simulink library "ddm"  (R2021b)
settings: Solver=VariableStepAuto  StartTime=0.0  StopTime=10.0  RelTol=1e-3
undefined symbols (not defined in the file or in its folder): ADDM_FrTMTqDev_X_Nm, ADDM_RrTMTqDev_X_Nm, ENUM_ADASACCSTA_ERROR, ENUM_ADASACCSTA_OFF, ENUM_ADASACCSTA_STANDBY, ENUM_ALLOWMOV_ALLOWREADY, ENUM_APS, ENUM_BRKSTA_ERROR, ENUM_BRKSTA_OFF, ENUM_BRKSTA_ON, ENUM_BRKSW_INVALID, ENUM_BRKSW_OFF, ENUM_BRKSW_ON, ENUM_CHGPREACTERRSTA_OBCPRE, ENUM_DCDCFAULTSTA_ANYFAULTLV1, ENUM_DCDCFAULTSTA_ANYFAULTLV2, ENUM_DRIVETRAIN_AWD, ENUM_DRIVETRAIN_FWD, ENUM_DRIVETRAIN_RWD, ENUM_EDUDRTSTA_NORMAL, ENUM_EPBSTA_APPLIED, ENUM_EPBSTA_RELEASED, ENUM_GEARACTUALPOSN_INVALID, ENUM_GEARACTUALPOSN_P, ENUM_HVBATTREADYPRE_READY, ENUM_MCUWARN_LV0, ENUM_MCUWARN_LV1, ENUM_MCUWARN_LV2, ENUM_MCUWARN_LV3, ENUM_MCUWARN_NOERROR, ENUM_OBCFAULTSTA_ANYFAULT, ENUM_PAS_R2F2, ENUM_PDFAULT_BATTPDFAIL, ENUM_PDFAULT_DCDCDISABLE, ENUM_PDFAULT_MCUDISABLE, ENUM_PDFAULT_MCUDISCHRG, ENUM_POWERSTA_OFF, ENUM_POWERSTA_ON, ENUM_POWERSTA_READY, ENUM_POWERSTA_STANDBY, ENUM_PRESSINDI_LOW, ENUM_PUFAULT_BATTUPFAIL, ENUM_PUFAULT_DCDCENABLEFAIL, ENUM_PUFAULT_PRECHRGCHKFAIL, ENUM_PUFAULT_SAFETYCHKFAIL, ENUM_PUSTATE_COMPLETED, ENUM_PWRSTASW_OFF, ENUM_PWRSTASW_OFFA, ENUM_PWRSTASW_OFFCHVCHRG, ENUM_PWRSTASW_OFFCLVCHRG, ENUM_PWRSTASW_ON, ENUM_PWRSTASW_ONHVCHRG, ENUM_PWRSTASW_READY, ENUM_PWRSTASW_STANDBY, ENUM_SHIFTCOMMAND_P, ENUM_SHIFTERERRSTA_PBUTTONFAILURE, ENUM_VEHMALFUNLV_2ND, ENUM_VEHMALFUNLV_3RD, ENUM_VEHMALFUNLV_4TH, ENUM_VEHMALFUNLV_NORMAL ... (+459)
libraries: hcu_lib x515, simulink x3
(part 21 of 25)

== system ddm/DDM/DDM/PMM/SW failure/Tailgate switch failure ==
  note: Diagnostics and Fault Handling
  note: Release Condition After Decision
  note: Test Detection Criteria
  note: Test Pass Criteria
  task_time_s : Inport
  VPMM_PowerSta_enum : Inport  Port=2
  VPMM_PwrStaSW_enum : Inport  Port=3
  VINP_TailgaSW : Inport  Port=4
  DTC_clear_request : Inport  Port=5
  Constant1 : Constant  Value=KDDM_TailgaSWDTC_cnt
  Constant11 : Constant  Value=KDDM_TailgaSWPassTO_s
  Constant12 : Constant  Value=ENUM_POWERSTA_STANDBY
  Constant13 : Constant  Value=ZERO_INT
  Constant15 : Constant  Value=KDDM_TailgaSWPassTO_s
  Constant16 : Constant  Value=KDDM_TailgaSWDetTO_s
  Constant17 : Constant  Value=KDDM_TailgaSW_s
  Constant18 : Constant  Value=FALSE
  Constant19 : Constant  Value=ENUM_PWRSTASW_OFF
  Constant2 : Constant  Value=KDDM_SWFailDiagnosisOffSW_flg
  Constant21 : Constant  Value=ZERO_INT
  Constant22 : Constant  Value=ENUM_PWRSTASW_OFF
  Constant23 : Constant  Value=TRUE
  Constant24 : Constant  Value=KDDM_TailgaSWPassTO_s
  Constant25 : Constant  Value=KDDM_TailgaSWDTC_cnt
  Constant26 : Constant  Value=ONE_INT
  Constant3 : Constant  Value=FALSE
  Constant32 : Constant  Value=ZERO_FLOAT
  Constant33 : Constant  Value=ENUM_POWERSTA_OFF
  Constant4 : Constant  Value=TRUE
  DTC_Couter2 : hcu_lib/Basic_Blocks/DTC_Couter
  DTC_Info : hcu_lib/Basic_Blocks/DTC_Info
  Data Type Conversion12 : DataTypeConversion  OutDataTypeStr=boolean
  Data Type Conversion14 : DataTypeConversion  OutDataTypeStr=boolean
  Data Type Conversion7 : DataTypeConversion
  Equal1 : RelationalOperator  Operator=~=  OutDataTypeStr=boolean  RndMeth=Simplest
  Equal11 : RelationalOperator  Operator===  OutDataTypeStr=boolean  RndMeth=Simplest
  Equal12 : RelationalOperator  Operator===  OutDataTypeStr=boolean  RndMeth=Simplest
  Equal3 : RelationalOperator  Operator=~=  OutDataTypeStr=boolean  RndMeth=Simplest
  Equal4 : RelationalOperator  Operator=~=  OutDataTypeStr=boolean  RndMeth=Simplest
  Equal5 : RelationalOperator  OutDataTypeStr=boolean  RndMeth=Simplest
  Logical Operator14 : Logic  Operator=OR  Inputs=4  AllPortsSameDT=off  OutDataTypeStr=boolean
  Logical Operator16 : Logic  AllPortsSameDT=off  OutDataTypeStr=boolean
  Logical Operator4 : Logic  Operator=NOT  AllPortsSameDT=off  OutDataTypeStr=boolean
  Logical Operator5 : Logic  Operator=NOT  AllPortsSameDT=off  OutDataTypeStr=boolean
  Logical Operator6 : Logic  AllPortsSameDT=off  OutDataTypeStr=boolean
  Logical Operator7 : Logic  Operator=NOT  AllPortsSameDT=off  OutDataTypeStr=boolean
  Relational Operator1 : RelationalOperator  Operator=>  OutDataTypeStr=boolean  RndMeth=Simplest
  Relational Operator4 : RelationalOperator  Operator=<=  OutDataTypeStr=boolean  RndMeth=Simplest
  Relational Operator5 : RelationalOperator  Operator=>  OutDataTypeStr=boolean  RndMeth=Simplest
  SR_Latch1 : hcu_lib/Basic_Blocks/SR_Latch
  Subsystem : Subsystem  AncestorBlock=ddm1/DDM/DDM/PMM/SW failure/Driver seat switch failure/Subsystem
  Switch{1,5,10,14} (4 alike) : Switch  Criteria=u2 ~= 0
  Terminator : Terminator
  Test Detection Criteria2 : hcu_lib/Basic_Blocks/Test Detection Criteria
  Timer : hcu_lib/Basic_Blocks/Test Detection Criteria/Timer
  Timer1 : hcu_lib/Basic_Blocks/Timer
  Unit Delay : UnitDelay  SampleTime=-1  HasFrameUpgradeWarning=on
  Unit Delay1 : UnitDelay  SampleTime=-1  HasFrameUpgradeWarning=on
  Unit Delay9 : UnitDelay  SampleTime=-1  HasFrameUpgradeWarning=on
  VDDM_TailgaSWDTC_raw32 : Outport
  VDDM_VCUTailgateSWSta_flg : Outport  Port=2
  VDDM_TailgaSWCFS_flg : Outport  Port=3
  wires:
  Switch1/1 -> VDDM_VCUTailgateSWSta_flg/1  "VDDM_VCUTailgateSWSta_flg"
  Constant3/1 -> Switch1/3
  [VDDM_TailgaSWCFS_flg] -> VDDM_TailgaSWCFS_flg/1, Switch1/2
  Constant4/1 -> Switch1/1
  Logical Operator14/1 -> [VDDM_TailgaSWCFSRls_flg]  "VDDM_TailgaSWCFSRls_flg"
  [VDDM_TailgaSWPass_flg] -> Logical Operator14/3
  Constant1/1 -> DTC_Couter2/3
  Relational Operator1/1 -> Terminator/1  "VDDM_TailgaSWDFS_flg"
  DTC_Couter2/2 -> Relational Operator1/1  "VDDM_TailgaSWDTC_cnt"
  Equal12/1 -> Logical Operator16/2
  DTC_Couter2/1 -> [VDDM_TailgaSWCFS_flg]  "VDDM_TailgaSWCFS_flg"
  Logical Operator16/1 -> Logical Operator14/1
  Equal11/1 -> Logical Operator16/1
  Constant13/1 -> Relational Operator1/2
  Constant2/1 -> Logical Operator14/4
  Constant12/1 -> Equal12/2
  [VDDM_TailgaSWCFSRls_flg] -> DTC_Couter2/2
  Unit Delay1/1 -> Equal11/1
  [DTC_clear_request] -> Logical Operator14/2
  Constant33/1 -> Equal11/2
  [VPMM_PowerSta_enum] -> Equal12/1
  [VPMM_PowerSta_enum] -> Unit Delay1/1
  [VDDM_TailgaSWDet_flg] -> DTC_Couter2/1
  Equal4/1 -> [VDDM_TailgaSWChange_flg]
  Data Type Conversion12/1 -> Test Detection Criteria2/1
  Subsystem/1(Fault_flg) -> Logical Operator6/1
  [VDDM_TailgaSWChange_flg] -> SR_Latch1/2
  Logical Operator7/1 -> Timer1/1
  [TailgaSWFault_flg] -> Switch10/1
  Data Type Conversion7/1 -> Test Detection Criteria2/4
  Test Detection Criteria2/1 -> [VDDM_TailgaSWDet_flg]  "VDDM_TailgaSWDet_flg"
  Constant26/1 -> SR_Latch1/1
  Switch5/1 -> Data Type Conversion12/1
  Constant32/1 -> Relational Operator5/2
  Switch10/1 -> Timer1/2, Logical Operator7/1
  Logical Operator6/1 -> Switch14/1, [TailgaSWFault_flg]
  [VPMM_PwrStaSW_enum] -> Equal1/1
  Relational Operator4/1 -> Logical Operator6/2
  [task_time_s] -> Timer1/3
  [task_time_s] -> Timer/3
  Constant21/1 -> Switch14/3
  Constant22/1 -> Equal1/2
  Data Type Conversion14/1 -> Equal4/1
  SR_Latch1/1 -> Timer/1, Logical Operator4/1, Logical Operator5/1
  Constant23/1 -> Switch10/3
  Logical Operator5/1 -> Subsystem/Trigger
  Constant17/1 -> Relational Operator4/2
  Constant24/1 -> Equal5/2
  [VINP_TailgaSWGPIO_flg] -> Relational Operator5/1
  Constant11/1 -> Timer/4
  Unit Delay/1 -> Subsystem/1(In1)
  Logical Operator4/1 -> Timer/2
  Relational Operator5/1 -> Equal4/2, Unit Delay9/1
  [task_time_s] -> Test Detection Criteria2/2
  [VDDM_TailgaSWCFSRls_flg] -> Switch5/2
  Constant18/1 -> Switch5/1
  Constant25/1 -> Test Detection Criteria2/3
  Equal5/1 -> [VDDM_TailgaSWPass_flg]  "VDDM_TailgaSWPass_flg"
  Timer1/1 -> Equal5/1
  Constant16/1 -> Data Type Conversion7/1
  Timer/1 -> Unit Delay/1, Relational Operator4/1
  Constant15/1 -> Timer1/4
  Unit Delay9/1 -> Data Type Conversion14/1
  Equal3/1 -> Switch10/2
  Switch14/1 -> Switch5/3
  Equal1/1 -> Switch14/2
  [VPMM_PwrStaSW_enum] -> Equal3/1
  Constant19/1 -> Equal3/2
  DTC_clear_request/1 -> [DTC_clear_request]
  VINP_TailgaSW/1 -> [VINP_TailgaSWGPIO_flg]
  task_time_s/1 -> [task_time_s]
  VPMM_PwrStaSW_enum/1 -> [VPMM_PwrStaSW_enum]
  VPMM_PowerSta_enum/1 -> [VPMM_PowerSta_enum]
  DTC_Info/1 -> VDDM_TailgaSWDTC_raw32/1  "VDDM_TailgaSWDTC_raw32"
  [VDDM_TailgaSWPass_flg] -> DTC_Info/2
  [VDDM_TailgaSWCFS_flg] -> DTC_Info/3
  [VDDM_TailgaSWDet_flg] -> DTC_Info/1
  [DTC_clear_request] -> DTC_Info/4

== system ddm/DDM/DDM/PMM/power up and power down/BMS HV relay closed fail ==
  note: Test Detection Criteria
  note: Test Pass Criteria
  note: Diagnostics and Fault Handling
  note: Release Condition After Decision
  task_time_s : Inport
  VPMM_PowerSta_enum : Inport  Port=2
  VPMM_PwrStaSW_enum : Inport  Port=3
  VINP_HVBContactorSta_flg : Inport  Port=4
  VPMM_PowerUpFault_enum : Inport  Port=5
  DTC_clear_request : Inport  Port=6
  VPMM_PowerUpState_enum : Inport  Port=7
  Constant : Constant  Value=ENUM_PUFAULT_BATTUPFAIL
  Constant12 : Constant  Value=ENUM_PWRSTASW_OFF
  Constant13 : Constant  Value=FALSE
  Constant14 : Constant  Value=ZERO_INT
  Constant17 : Constant  Value=KDDM_PwrUpDnDiagnosisOffSW_flg
  Constant18 : Constant  Value=KDDM_HVRlyCloDTC_cnt
  Constant22 : Constant  Value=ENUM_POWERSTA_OFF
  Constant28 : Constant  Value=KDDM_HVRlyCloDTC_cnt
  Constant29 : Constant  Value=FALSE
  Constant3 : Constant  Value=KDDM_HVRlyCloPassTO_s
  Constant4 : Constant  Value=FALSE
  Constant41 : Constant  Value=KDDM_HVRlyCloDetTO_s
  Constant5 : Constant  Value=ENUM_PUSTATE_COMPLETED
  Constant6 : Constant  Value=TRUE
  Constant7 : Constant  Value=ENUM_POWERSTA_STANDBY
  Constant9 : Constant  Value=KDDM_HVRlyCloPassTO_s
  DTC_Couter1 : hcu_lib/Basic_Blocks/DTC_Couter
  DTC_Info : hcu_lib/Basic_Blocks/DTC_Info
  Equal{1,3,8..9} (4 alike) : RelationalOperator  Operator===  OutDataTypeStr=boolean  RndMeth=Simplest
  Equal4 : RelationalOperator  Operator=~=  OutDataTypeStr=boolean  RndMeth=Simplest
  Equal7 : RelationalOperator  OutDataTypeStr=boolean  RndMeth=Simplest
  Logical Operator13 : Logic  Operator=NOT  AllPortsSameDT=off  OutDataTypeStr=boolean
  Logical Operator14 : Logic  Operator=OR  Inputs=4  AllPortsSameDT=off  OutDataTypeStr=boolean
  Logical Operator16 : Logic  AllPortsSameDT=off  OutDataTypeStr=boolean
  Logical Operator4 : Logic  Operator=NOT  AllPortsSameDT=off  OutDataTypeStr=boolean
  Logical Operator5 : Logic  AllPortsSameDT=off  OutDataTypeStr=boolean
  Relational Operator1 : RelationalOperator  Operator=>  OutDataTypeStr=boolean  RndMeth=Simplest
  Switch1 : Switch  Criteria=u2 ~= 0
  Switch3 : Switch  Criteria=u2 ~= 0
  Switch6 : Switch  Criteria=u2 ~= 0
  Terminator : Terminator
  Test Detection Criteria1 : hcu_lib/Basic_Blocks/Test Detection Criteria
  Timer2 : hcu_lib/Basic_Blocks/Timer
  Unit Delay1 : UnitDelay  SampleTime=-1  HasFrameUpgradeWarning=on
  VDDM_HVRlyCloDTC_raw32 : Outport
  VDDM_HVRlyCloCFS_flg : Outport  Port=2
  wires:
  [VDDM_HVRlyCloCFS_flg] -> VDDM_HVRlyCloCFS_flg/1
  DTC_Couter1/1 -> [VDDM_HVRlyCloCFS_flg]  "VDDM_HVRlyCloCFS_flg"
  [VPMM_PwrStaSW_enum] -> Equal4/1
  Equal7/1 -> [VDDM_HVRlyCloPass_flg]  "VDDM_HVRlyCloPass_flg"
  [task_time_s] -> Test Detection Criteria1/2
  Constant28/1 -> Test Detection Criteria1/3
  Unit Delay1/1 -> Equal8/1
  [VDDM_HVRlyCloChk_flg] -> Switch3/1
  Test Detection Criteria1/1 -> [VDDM_HVRlyCloDet_flg]  "VDDM_HVRlyCloDet_flg"
  Equal9/1 -> Logical Operator16/2
  DTC_Couter1/2 -> Relational Operator1/1  "VDDM_HVRlyCloDTC_cnt"
  Switch6/1 -> Test Detection Criteria1/1
  Constant3/1 -> Timer2/4
  Constant5/1 -> Equal3/2
  Switch1/1 -> Logical Operator13/1, Timer2/2
  Logical Operator14/1 -> [VDDM_HVRlyCloCFSRls_flg]  "VDDM_HVRlyCloCFSRls_flg"
  Switch3/1 -> Switch6/3
  Constant6/1 -> Switch1/3
  Constant13/1 -> Switch3/3
  Constant14/1 -> Relational Operator1/2
  [VDDM_HVRlyCloPass_flg] -> Logical Operator14/3
  [DTC_clear_request] -> Logical Operator14/2
  Constant29/1 -> Switch6/1
  Equal4/1 -> Switch3/2
  Constant9/1 -> Equal7/2
  [VDDM_HVRlyCloCFSRls_flg] -> DTC_Couter1/2
  Constant41/1 -> Test Detection Criteria1/4
  Logical Operator16/1 -> Logical Operator14/1
  Constant12/1 -> Equal4/2
  Logical Operator13/1 -> Timer2/1
  Equal8/1 -> Logical Operator16/1
  Equal3/1 -> Switch1/2
  [VPMM_PowerUpState_enum] -> Equal3/1
  Timer2/1 -> Equal7/1
  Constant18/1 -> DTC_Couter1/3
  Constant17/1 -> Logical Operator14/4
  [VPMM_PowerSta_enum] -> Unit Delay1/1
  [VPMM_PowerSta_enum] -> Equal9/1
  Constant22/1 -> Equal8/2
  Constant7/1 -> Equal9/2
  [task_time_s] -> Timer2/3
  Constant4/1 -> Switch1/1
  [VDDM_HVRlyCloDet_flg] -> DTC_Couter1/1
  Relational Operator1/1 -> Terminator/1  "VDDM_HVRlyCloDFS_flg"
  [VDDM_HVRlyCloCFSRls_flg] -> Switch6/2
  task_time_s/1 -> [task_time_s]
  VPMM_PwrStaSW_enum/1 -> [VPMM_PwrStaSW_enum]
  VPMM_PowerSta_enum/1 -> [VPMM_PowerSta_enum]
  DTC_clear_request/1 -> [DTC_clear_request]
  Constant/1 -> Equal1/2
  Equal1/1 -> Logical Operator5/2
  Logical Operator4/1 -> Logical Operator5/1
  VINP_HVBContactorSta_flg/1 -> Logical Operator4/1
  VPMM_PowerUpFault_enum/1 -> Equal1/1
  Logical Operator5/1 -> [VDDM_HVRlyCloChk_flg]
  DTC_Info/1 -> VDDM_HVRlyCloDTC_raw32/1  "VDDM_HVRlyCloDTC_raw32"
  [VDDM_HVRlyCloPass_flg] -> DTC_Info/2
  [VDDM_HVRlyCloCFS_flg] -> DTC_Info/3
  [VDDM_HVRlyCloDet_flg] -> DTC_Info/1
  [DTC_clear_request] -> DTC_Info/4
  VPMM_PowerUpState_enum/1 -> [VPMM_PowerUpState_enum]

== system ddm/DDM/DDM/PMM/power up and power down/BMS HV relay opened fail ==
  note: Test Detection Criteria
  note: Diagnostics and Fault Handling
  note: Test Pass Criteria
  note: Release Condition After Decision
  task_time_s : Inport
  VPMM_PowerSta_enum : Inport  Port=2
  VPMM_PwrStaSW_enum : Inport  Port=3
  VPMM_PowerDownFault_enum : Inport  Port=4
  DTC_clear_request : Inport  Port=5
  Constant : Constant  Value=ENUM_PDFAULT_BATTPDFAIL
  Constant1 : Constant  Value=FALSE
  Constant12 : Constant  Value=ENUM_PWRSTASW_OFF
  Constant13 : Constant  Value=FALSE
  Constant14 : Constant  Value=ZERO_INT
  Constant18 : Constant  Value=KDDM_HVRlyOpDTC_cnt
  Constant19 : Constant  Value=KDDM_HVRlyOpDTC_cnt
  Constant2 : Constant  Value=TRUE
  Constant29 : Constant  Value=FALSE
  Constant3 : Constant  Value=KDDM_PwrUpDnDiagnosisOffSW_flg
  Constant4 : Constant  Value=ENUM_POWERSTA_OFF
  Constant41 : Constant  Value=KDDM_HVRlyOpDetTO_s
  Constant5 : Constant  Value=ENUM_PWRSTASW_OFF
  Constant6 : Constant  Value=TRUE
  Constant7 : Constant  Value=KDDM_HVRlyOpPassTO_s
  Constant8 : Constant  Value=KDDM_HVRlyOpPassTO_s
  Constant9 : Constant  Value=ENUM_POWERSTA_STANDBY
  DTC_Couter1 : hcu_lib/Basic_Blocks/DTC_Couter
  DTC_Info : hcu_lib/Basic_Blocks/DTC_Info
  Equal1 : RelationalOperator  Operator===  OutDataTypeStr=boolean  RndMeth=Simplest
  Equal10 : RelationalOperator  Operator===  OutDataTypeStr=boolean  RndMeth=Simplest
  Equal3 : RelationalOperator  Operator=~=  OutDataTypeStr=boolean  RndMeth=Simplest
  Equal5 : RelationalOperator  Operator=~=  OutDataTypeStr=boolean  RndMeth=Simplest
  Equal8 : RelationalOperator  OutDataTypeStr=boolean  RndMeth=Simplest
  Equal9 : RelationalOperator  Operator===  OutDataTypeStr=boolean  RndMeth=Simplest
  Logical Operator13 : Logic  Operator=NOT  AllPortsSameDT=off  OutDataTypeStr=boolean
  Logical Operator14 : Logic  Operator=OR  Inputs=4  AllPortsSameDT=off  OutDataTypeStr=boolean
  Logical Operator16 : Logic  AllPortsSameDT=off  OutDataTypeStr=boolean
  Relational Operator1 : RelationalOperator  Operator=>  OutDataTypeStr=boolean  RndMeth=Simplest
  Switch{1..3,6} (4 alike) : Switch  Criteria=u2 ~= 0
  Terminator : Terminator
  Test Detection Criteria1 : hcu_lib/Basic_Blocks/Test Detection Criteria
  Timer2 : hcu_lib/Basic_Blocks/Timer
  Unit Delay1 : UnitDelay  SampleTime=-1  HasFrameUpgradeWarning=on
  VDDM_HVRlyOpDTC_raw32 : Outport
  VDDM_HVRlyOpFail_flg : Outport  Port=2
  VDDM_HVRlyOpCFS_flg : Outport  Port=3
  wires:
  Constant1/1 -> Switch1/3
  Constant2/1 -> Switch1/1
  Switch1/1 -> VDDM_HVRlyOpFail_flg/1  "VDDM_HVRlyOpFail_flg"
  [VDDM_HVRlyOpPass_flg] -> Logical Operator14/3
  Constant5/1 -> Equal3/2
  Constant6/1 -> Switch2/3
  Equal3/1 -> Switch2/2
  [VPMM_PwrStaSW_enum] -> Equal3/1
  [VDDM_HVRlyOpChk_flg] -> Switch2/1
  Constant8/1 -> Equal8/2
  DTC_Couter1/2 -> Relational Operator1/1  "VDDM_HVRlyOpDTC_cnt"
  [VDDM_HVRlyOpCFSRls_flg] -> Switch6/2
  Logical Operator13/1 -> Timer2/1
  [task_time_s] -> Timer2/3
  Constant18/1 -> DTC_Couter1/3
  [VDDM_HVRlyOpChk_flg] -> Switch3/1
  [VDDM_HVRlyOpDet_flg] -> DTC_Couter1/1
  Constant7/1 -> Timer2/4
  Relational Operator1/1 -> Terminator/1  "VDDM_HVRlyOpDFS_flg"
  Switch2/1 -> Logical Operator13/1, Timer2/2
  Test Detection Criteria1/1 -> [VDDM_HVRlyOpDet_flg]  "VDDM_HVRlyOpDet_flg"
  Switch3/1 -> Switch6/3
  [VDDM_HVRlyOpCFSRls_flg] -> DTC_Couter1/2
  Constant9/1 -> Equal10/2
  Unit Delay1/1 -> Equal9/1
  [VPMM_PowerSta_enum] -> Equal10/1
  Constant41/1 -> Test Detection Criteria1/4
  [VPMM_PowerSta_enum] -> Unit Delay1/1
  [DTC_clear_request] -> Logical Operator14/2
  Constant4/1 -> Equal9/2
  Logical Operator16/1 -> Logical Operator14/1
  Timer2/1 -> Equal8/1
  Equal9/1 -> Logical Operator16/1
  Constant12/1 -> Equal5/2
  Constant3/1 -> Logical Operator14/4
  Constant29/1 -> Switch6/1
  DTC_Couter1/1 -> [VDDM_HVRlyOpCFS_flg]  "VDDM_HVRlyOpCFS_flg"
  Equal5/1 -> Switch3/2
  Constant13/1 -> Switch3/3
  Constant14/1 -> Relational Operator1/2
  Equal10/1 -> Logical Operator16/2
  Switch6/1 -> Test Detection Criteria1/1
  [task_time_s] -> Test Detection Criteria1/2
  [VPMM_PwrStaSW_enum] -> Equal5/1
  Logical Operator14/1 -> [VDDM_HVRlyOpCFSRls_flg]  "VDDM_HVRlyOpCFSRls_flg"
  Equal8/1 -> [VDDM_HVRlyOpPass_flg]  "VDDM_HVRlyOpPass_flg"
  Constant19/1 -> Test Detection Criteria1/3
  task_time_s/1 -> [task_time_s]
  VPMM_PwrStaSW_enum/1 -> [VPMM_PwrStaSW_enum]
  VPMM_PowerSta_enum/1 -> [VPMM_PowerSta_enum]
  DTC_clear_request/1 -> [DTC_clear_request]
  VPMM_PowerDownFault_enum/1 -> Equal1/1
  Constant/1 -> Equal1/2
  Equal1/1 -> [VDDM_HVRlyOpChk_flg]
  [VDDM_HVRlyOpCFS_flg] -> VDDM_HVRlyOpCFS_flg/1, Switch1/2
  DTC_Info/1 -> VDDM_HVRlyOpDTC_raw32/1  "VDDM_HVRlyOpDTC_raw32"
  [VDDM_HVRlyOpPass_flg] -> DTC_Info/2
  [VDDM_HVRlyOpCFS_flg] -> DTC_Info/3
  [VDDM_HVRlyOpDet_flg] -> DTC_Info/1
  [DTC_clear_request] -> DTC_Info/4

== system ddm/DDM/DDM/PMM/power up and power down/BMS ready fail ==
  note: Test Pass Criteria
  note: Release Condition After Decision
  note: Diagnostics and Fault Handling
  note: Test Detection Criteria
  task_time_s : Inport
  VPMM_PowerSta_enum : Inport  Port=2
  VPMM_PwrStaSW_enum : Inport  Port=3
  VINP_BMSREADY_flg : Inport  Port=4
  VPMM_PowerUpFault_enum : Inport  Port=5
  DTC_clear_request : Inport  Port=6
  VPMM_PowerUpState_enum : Inport  Port=7
  Constant : Constant  Value=ENUM_PUFAULT_BATTUPFAIL
  Constant12 : Constant  Value=ENUM_PWRSTASW_OFF
  Constant13 : Constant  Value=FALSE
  Constant14 : Constant  Value=ZERO_INT
  Constant17 : Constant  Value=KDDM_PwrUpDnDiagnosisOffSW_flg
  Constant18 : Constant  Value=KDDM_BMSRdyPassTO_s
  Constant22 : Constant  Value=ENUM_POWERSTA_OFF
  Constant26 : Constant  Value=KDDM_BMSRdyDTC_cnt
  Constant28 : Constant  Value=KDDM_BMSRdyDTC_cnt
  Constant29 : Constant  Value=FALSE
  Constant4 : Constant  Value=FALSE
  Constant41 : Constant  Value=KDDM_BMSRdyDetTO_s
  Constant5 : Constant  Value=ENUM_PUSTATE_COMPLETED
  Constant6 : Constant  Value=TRUE
  Constant7 : Constant  Value=ENUM_POWERSTA_STANDBY
  Constant9 : Constant  Value=KDDM_BMSRdyPassTO_s
  DTC_Couter1 : hcu_lib/Basic_Blocks/DTC_Couter
  DTC_Info : hcu_lib/Basic_Blocks/DTC_Info
  Equal{1,3,8..9} (4 alike) : RelationalOperator  Operator===  OutDataTypeStr=boolean  RndMeth=Simplest
  Equal4 : RelationalOperator  Operator=~=  OutDataTypeStr=boolean  RndMeth=Simplest
  Equal7 : RelationalOperator  OutDataTypeStr=boolean  RndMeth=Simplest
  Logical Operator13 : Logic  Operator=NOT  AllPortsSameDT=off  OutDataTypeStr=boolean
  Logical Operator14 : Logic  Operator=OR  Inputs=4  AllPortsSameDT=off  OutDataTypeStr=boolean
  Logical Operator16 : Logic  AllPortsSameDT=off  OutDataTypeStr=boolean
  Logical Operator4 : Logic  Operator=NOT  AllPortsSameDT=off  OutDataTypeStr=boolean
  Logical Operator5 : Logic  AllPortsSameDT=off  OutDataTypeStr=boolean
  Relational Operator1 : RelationalOperator  Operator=>  OutDataTypeStr=boolean  RndMeth=Simplest
  Switch1 : Switch  Criteria=u2 ~= 0
  Switch3 : Switch  Criteria=u2 ~= 0
  Switch6 : Switch  Criteria=u2 ~= 0
  Terminator : Terminator
  Test Detection Criteria1 : hcu_lib/Basic_Blocks/Test Detection Criteria
  Timer2 : hcu_lib/Basic_Blocks/Timer
  Unit Delay1 : UnitDelay  SampleTime=-1  HasFrameUpgradeWarning=on
  VDDM_BMSRdyDTC_raw32 : Outport
  VDDM_BMSRdyCFS_flg : Outport  Port=2
  wires:
  [VDDM_BMSRdyCFS_flg] -> VDDM_BMSRdyCFS_flg/1
  Constant12/1 -> Equal4/2
  Constant9/1 -> Timer2/4
  [VPMM_PwrStaSW_enum] -> Equal4/1
  Timer2/1 -> Equal7/1
  Switch1/1 -> Logical Operator13/1, Timer2/2
  Constant6/1 -> Switch1/3
  Constant22/1 -> Equal8/2
  Logical Operator16/1 -> Logical Operator14/1
  Equal8/1 -> Logical Operator16/1
  Constant14/1 -> Relational Operator1/2
  Constant28/1 -> Test Detection Criteria1/3
  Constant18/1 -> Equal7/2
  [task_time_s] -> Timer2/3
  Constant41/1 -> Test Detection Criteria1/4
  [VPMM_PowerUpState_enum] -> Equal3/1
  [VDDM_BMSRdyCFSRls_flg] -> DTC_Couter1/2
  Constant26/1 -> DTC_Couter1/3
  Logical Operator13/1 -> Timer2/1
  Relational Operator1/1 -> Terminator/1  "VDDM_BMSRdyDFS_flg"
  DTC_Couter1/2 -> Relational Operator1/1  "VDDM_BMSRdyDTC_cnt"
  [VDDM_BMSRdyDet_flg] -> DTC_Couter1/1
  Constant4/1 -> Switch1/1
  Equal9/1 -> Logical Operator16/2
  Switch6/1 -> Test Detection Criteria1/1
  Constant17/1 -> Logical Operator14/4
  [task_time_s] -> Test Detection Criteria1/2
  Unit Delay1/1 -> Equal8/1
  Constant5/1 -> Equal3/2
  Constant7/1 -> Equal9/2
  Constant29/1 -> Switch6/1
  Constant13/1 -> Switch3/3
  Logical Operator14/1 -> [VDDM_BMSRdyCFSRls_flg]  "VDDM_BMSRdyCFSRls_flg"
  [VDDM_BMSRdyPass_flg] -> Logical Operator14/3
  Test Detection Criteria1/1 -> [VDDM_BMSRdyDet_flg]  "VDDM_BMSRdyDet_flg"
  Equal4/1 -> Switch3/2
  [VPMM_PowerSta_enum] -> Equal9/1
  Switch3/1 -> Switch6/3
  [VDDM_BMSRdyCFSRls_flg] -> Switch6/2
  [VPMM_PowerSta_enum] -> Unit Delay1/1
  DTC_Couter1/1 -> [VDDM_BMSRdyCFS_flg]  "VDDM_BMSRdyCFS_flg"
  [VDDM_BMSRdyChk_flg] -> Switch3/1
  Equal7/1 -> [VDDM_BMSRdyPass_flg]  "VDDM_BMSRdyPass_flg"
  [DTC_clear_request] -> Logical Operator14/2
  Equal3/1 -> Switch1/2
  Logical Operator5/1 -> [VDDM_BMSRdyChk_flg]
  VPMM_PowerUpFault_enum/1 -> Equal1/1
  VINP_BMSREADY_flg/1 -> Logical Operator4/1
  Logical Operator4/1 -> Logical Operator5/1
  Equal1/1 -> Logical Operator5/2
  Constant/1 -> Equal1/2
  DTC_clear_request/1 -> [DTC_clear_request]
  VPMM_PowerSta_enum/1 -> [VPMM_PowerSta_enum]
  VPMM_PwrStaSW_enum/1 -> [VPMM_PwrStaSW_enum]
  task_time_s/1 -> [task_time_s]
  DTC_Info/1 -> VDDM_BMSRdyDTC_raw32/1  "VDDM_BMSRdyDTC_raw32"
  [VDDM_BMSRdyCFS_flg] -> DTC_Info/3
  [VDDM_BMSRdyDet_flg] -> DTC_Info/1
  [VDDM_BMSRdyPass_flg] -> DTC_Info/2
  [DTC_clear_request] -> DTC_Info/4
  VPMM_PowerUpState_enum/1 -> [VPMM_PowerUpState_enum]

== system ddm/DDM/DDM/PMM/power up and power down/DCDC disable fail ==
  note: Release Condition After Decision
  note: Test Detection Criteria
  note: Diagnostics and Fault Handling
  note: Test Pass Criteria
  task_time_s : Inport
  VPMM_PowerSta_enum : Inport  Port=2
  VPMM_PwrStaSW_enum : Inport  Port=3
  VPMM_PowerDownFault_enum : Inport  Port=4
  DTC_clear_request : Inport  Port=5
  Constant : Constant  Value=ENUM_PDFAULT_DCDCDISABLE
  Constant1 : Constant  Value=ENUM_PWRSTASW_OFF
  Constant12 : Constant  Value=ENUM_PWRSTASW_OFF
  Constant13 : Constant  Value=FALSE
  Constant14 : Constant  Value=ZERO_INT
  Constant18 : Constant  Value=KDDM_DCDCDisDTC_cnt
  Constant2 : Constant  Value=KDDM_PwrUpDnDiagnosisOffSW_flg
  Constant23 : Constant  Value=TRUE
  Constant26 : Constant  Value=KDDM_DCDCDisDTC_cnt
  Constant29 : Constant  Value=FALSE
  Constant3 : Constant  Value=ENUM_POWERSTA_OFF
  Constant4 : Constant  Value=KDDM_DCDCDisPassTO_s
  Constant41 : Constant  Value=KDDM_DCDCDisDetTO_s
  Constant8 : Constant  Value=ENUM_POWERSTA_STANDBY
  Constant9 : Constant  Value=KDDM_DCDCDisPassTO_s
  DTC_Couter1 : hcu_lib/Basic_Blocks/DTC_Couter
  DTC_Info : hcu_lib/Basic_Blocks/DTC_Info
  Equal1 : RelationalOperator  Operator===  OutDataTypeStr=boolean  RndMeth=Simplest
  Equal10 : RelationalOperator  Operator===  OutDataTypeStr=boolean  RndMeth=Simplest
  Equal2 : RelationalOperator  Operator=~=  OutDataTypeStr=boolean  RndMeth=Simplest
  Equal5 : RelationalOperator  Operator=~=  OutDataTypeStr=boolean  RndMeth=Simplest
  Equal8 : RelationalOperator  OutDataTypeStr=boolean  RndMeth=Simplest
  Equal9 : RelationalOperator  Operator===  OutDataTypeStr=boolean  RndMeth=Simplest
  Logical Operator13 : Logic  Operator=NOT  AllPortsSameDT=off  OutDataTypeStr=boolean
  Logical Operator14 : Logic  Operator=OR  Inputs=4  AllPortsSameDT=off  OutDataTypeStr=boolean
  Logical Operator16 : Logic  AllPortsSameDT=off  OutDataTypeStr=boolean
  Relational Operator1 : RelationalOperator  Operator=>  OutDataTypeStr=boolean  RndMeth=Simplest
  Switch1 : Switch  Criteria=u2 ~= 0
  Switch3 : Switch  Criteria=u2 ~= 0
  Switch6 : Switch  Criteria=u2 ~= 0
  Terminator : Terminator
  Test Detection Criteria1 : hcu_lib/Basic_Blocks/Test Detection Criteria
  Timer2 : hcu_lib/Basic_Blocks/Timer
  Unit Delay1 : UnitDelay  SampleTime=-1  HasFrameUpgradeWarning=on
  VDDM_DCDCDisDTC_raw32 : Outport
  VDDM_DCDCDisCFS_flg : Outport  Port=2
  wires:
  [VDDM_DCDCDisCFS_flg] -> VDDM_DCDCDisCFS_flg/1
  Constant1/1 -> Equal2/2
  Constant23/1 -> Switch1/3
  [VPMM_PwrStaSW_enum] -> Equal2/1
  Equal2/1 -> Switch1/2
  [VDDM_DCDCDisChk_flg] -> Switch1/1
  Constant18/1 -> DTC_Couter1/3
  Timer2/1 -> Equal8/1
  [VPMM_PwrStaSW_enum] -> Equal5/1
  [VDDM_DCDCDisPass_flg] -> Logical Operator14/3
  [VDDM_DCDCDisCFSRls_flg] -> Switch6/2
  Equal9/1 -> Logical Operator16/1
  Constant26/1 -> Test Detection Criteria1/3
  Equal8/1 -> [VDDM_DCDCDisPass_flg]  "VDDM_DCDCDisPass_flg"
  Switch1/1 -> Logical Operator13/1, Timer2/2
  Switch6/1 -> Test Detection Criteria1/1
  Constant41/1 -> Test Detection Criteria1/4
  DTC_Couter1/2 -> Relational Operator1/1  "VDDM_DCDCDisDTC_cnt"
  Equal10/1 -> Logical Operator16/2
  [VDDM_DCDCDisCFSRls_flg] -> DTC_Couter1/2
  Unit Delay1/1 -> Equal9/1
  Constant12/1 -> Equal5/2
  Test Detection Criteria1/1 -> [VDDM_DCDCDisDet_flg]  "VDDM_DCDCDisDet_flg"
  [task_time_s] -> Test Detection Criteria1/2
  [VDDM_DCDCDisDet_flg] -> DTC_Couter1/1
  [task_time_s] -> Timer2/3
  [VPMM_PowerSta_enum] -> Unit Delay1/1
  Constant2/1 -> Logical Operator14/4
  [VPMM_PowerSta_enum] -> Equal10/1
  Constant8/1 -> Equal10/2
  Constant3/1 -> Equal9/2
  Logical Operator13/1 -> Timer2/1
  Logical Operator16/1 -> Logical Operator14/1
  Logical Operator14/1 -> [VDDM_DCDCDisCFSRls_flg]  "VDDM_DCDCDisCFSRls_flg"
  [VDDM_DCDCDisChk_flg] -> Switch3/1
  Relational Operator1/1 -> Terminator/1  "VDDM_DCDCDisDFS_flg"
  Switch3/1 -> Switch6/3
  Constant13/1 -> Switch3/3
  Equal5/1 -> Switch3/2
  Constant29/1 -> Switch6/1
  DTC_Couter1/1 -> [VDDM_DCDCDisCFS_flg]  "VDDM_DCDCDisCFS_flg"
  [DTC_clear_request] -> Logical Operator14/2
  Constant14/1 -> Relational Operator1/2
  Constant4/1 -> Timer2/4
  Constant9/1 -> Equal8/2
  VPMM_PowerSta_enum/1 -> [VPMM_PowerSta_enum]
  VPMM_PwrStaSW_enum/1 -> [VPMM_PwrStaSW_enum]
  task_time_s/1 -> [task_time_s]
  VPMM_PowerDownFault_enum/1 -> Equal1/1
  Constant/1 -> Equal1/2
  DTC_clear_request/1 -> [DTC_clear_request]
  Equal1/1 -> [VDDM_DCDCDisChk_flg]
  DTC_Info/1 -> VDDM_DCDCDisDTC_raw32/1  "VDDM_DCDCDisDTC_raw32"
  [VDDM_DCDCDisPass_flg] -> DTC_Info/2
  [VDDM_DCDCDisCFS_flg] -> DTC_Info/3
  [VDDM_DCDCDisDet_flg] -> DTC_Info/1
  [DTC_clear_request] -> DTC_Info/4

== system ddm/DDM/DDM/PMM/power up and power down/DCDC enable fail ==
  note: Release Condition After Decision
  note: Test Detection Criteria
  note: Test Pass Criteria
  note: Diagnostics and Fault Handling
  task_time_s : Inport
  VPMM_PowerSta_enum : Inport  Port=2
  VPMM_PwrStaSW_enum : Inport  Port=3
  VINP_DCDCEnabled_flg : Inport  Port=4
  VPMM_PowerUpFault_enum : Inport  Port=5
  DTC_clear_request : Inport  Port=6
  VPMM_PowerUpState_enum : Inport  Port=7
  Constant : Constant  Value=ENUM_PUFAULT_DCDCENABLEFAIL
  Constant12 : Constant  Value=ENUM_PWRSTASW_OFF
  Constant13 : Constant  Value=FALSE
  Constant14 : Constant  Value=ZERO_INT
  Constant17 : Constant  Value=KDDM_PwrUpDnDiagnosisOffSW_flg
  Constant18 : Constant  Value=KDDM_DCDCEnaDTC_cnt
  Constant22 : Constant  Value=ENUM_POWERSTA_OFF
  Constant28 : Constant  Value=KDDM_DCDCEnaDTC_cnt
  Constant29 : Constant  Value=FALSE
  Constant3 : Constant  Value=KDDM_DCDCEnaPassTO_s
  Constant4 : Constant  Value=FALSE
  Constant41 : Constant  Value=KDDM_DCDCEnaDetTO_s
  Constant5 : Constant  Value=ENUM_PUSTATE_COMPLETED
  Constant6 : Constant  Value=TRUE
  Constant7 : Constant  Value=ENUM_POWERSTA_STANDBY
  Constant9 : Constant  Value=KDDM_DCDCEnaPassTO_s
  DTC_Couter1 : hcu_lib/Basic_Blocks/DTC_Couter
  DTC_Info : hcu_lib/Basic_Blocks/DTC_Info
  Equal{1,3,8..9} (4 alike) : RelationalOperator  Operator===  OutDataTypeStr=boolean  RndMeth=Simplest
  Equal4 : RelationalOperator  Operator=~=  OutDataTypeStr=boolean  RndMeth=Simplest
  Equal7 : RelationalOperator  OutDataTypeStr=boolean  RndMeth=Simplest
  Logical Operator13 : Logic  Operator=NOT  AllPortsSameDT=off  OutDataTypeStr=boolean
  Logical Operator14 : Logic  Operator=OR  Inputs=4  AllPortsSameDT=off  OutDataTypeStr=boolean
  Logical Operator16 : Logic  AllPortsSameDT=off  OutDataTypeStr=boolean
  Logical Operator4 : Logic  Operator=NOT  AllPortsSameDT=off  OutDataTypeStr=boolean
  Logical Operator5 : Logic  AllPortsSameDT=off  OutDataTypeStr=boolean
  Relational Operator1 : RelationalOperator  Operator=>  OutDataTypeStr=boolean  RndMeth=Simplest
  Switch1 : Switch  Criteria=u2 ~= 0
  Switch3 : Switch  Criteria=u2 ~= 0
  Switch6 : Switch  Criteria=u2 ~= 0
  Terminator : Terminator
  Test Detection Criteria1 : hcu_lib/Basic_Blocks/Test Detection Criteria
  Timer2 : hcu_lib/Basic_Blocks/Timer
  Unit Delay1 : UnitDelay  SampleTime=-1  HasFrameUpgradeWarning=on
  VDDM_DCDCEnaDTC_raw32 : Outport
  VDDM_DCDCEnaCFS_flg : Outport  Port=2
  wires:
  [VDDM_DCDCEnaCFS_flg] -> VDDM_DCDCEnaCFS_flg/1
  Constant6/1 -> Switch1/3
  Logical Operator13/1 -> Timer2/1
  Logical Operator16/1 -> Logical Operator14/1
  Timer2/1 -> Equal7/1
  [VPMM_PwrStaSW_enum] -> Equal4/1
  Logical Operator14/1 -> [VDDM_DCDCEnaCFSRls_flg]  "VDDM_DCDCEnaCFSRls_flg"
  Equal8/1 -> Logical Operator16/1
  Constant18/1 -> DTC_Couter1/3
  [VPMM_PowerUpState_enum] -> Equal3/1
  Constant41/1 -> Test Detection Criteria1/4
  DTC_Couter1/2 -> Relational Operator1/1  "VDDM_DCDCEnaDTC_cnt"
  Relational Operator1/1 -> Terminator/1  "VDDM_DCDCEnaDFS_flg"
  [task_time_s] -> Timer2/3
  [VDDM_DCDCEnaChk_flg] -> Switch3/1
  [VPMM_PowerSta_enum] -> Unit Delay1/1
  Constant22/1 -> Equal8/2
  Constant28/1 -> Test Detection Criteria1/3
  Constant13/1 -> Switch3/3
  Switch6/1 -> Test Detection Criteria1/1
  DTC_Couter1/1 -> [VDDM_DCDCEnaCFS_flg]  "VDDM_DCDCEnaCFS_flg"
  Equal9/1 -> Logical Operator16/2
  [task_time_s] -> Test Detection Criteria1/2
  Constant3/1 -> Timer2/4
  Constant17/1 -> Logical Operator14/4
  Equal4/1 -> Switch3/2
  [VDDM_DCDCEnaCFSRls_flg] -> Switch6/2
  Unit Delay1/1 -> Equal8/1
  [VPMM_PowerSta_enum] -> Equal9/1
  Constant7/1 -> Equal9/2
  Constant29/1 -> Switch6/1
  Constant5/1 -> Equal3/2
  [VDDM_DCDCEnaPass_flg] -> Logical Operator14/3
  Constant12/1 -> Equal4/2
  [DTC_clear_request] -> Logical Operator14/2
  Switch1/1 -> Logical Operator13/1, Timer2/2
  Switch3/1 -> Switch6/3
  Constant14/1 -> Relational Operator1/2
  Constant9/1 -> Equal7/2
  Equal3/1 -> Switch1/2
  Constant4/1 -> Switch1/1
  Equal7/1 -> [VDDM_DCDCEnaPass_flg]  "VDDM_DCDCEnaPass_flg"
  [VDDM_DCDCEnaDet_flg] -> DTC_Couter1/1
  Test Detection Criteria1/1 -> [VDDM_DCDCEnaDet_flg]  "VDDM_DCDCEnaDet_flg"
  [VDDM_DCDCEnaCFSRls_flg] -> DTC_Couter1/2
  task_time_s/1 -> [task_time_s]
  VPMM_PwrStaSW_enum/1 -> [VPMM_PwrStaSW_enum]
  VPMM_PowerSta_enum/1 -> [VPMM_PowerSta_enum]
  DTC_clear_request/1 -> [DTC_clear_request]
  Constant/1 -> Equal1/2
  Equal1/1 -> Logical Operator5/2
  Logical Operator4/1 -> Logical Operator5/1
  VINP_DCDCEnabled_flg/1 -> Logical Operator4/1
  VPMM_PowerUpFault_enum/1 -> Equal1/1
  Logical Operator5/1 -> [VDDM_DCDCEnaChk_flg]
  DTC_Info/1 -> VDDM_DCDCEnaDTC_raw32/1  "VDDM_DCDCEnaDTC_raw32"
  [VDDM_DCDCEnaPass_flg] -> DTC_Info/2
  [VDDM_DCDCEnaCFS_flg] -> DTC_Info/3
  [VDDM_DCDCEnaDet_flg] -> DTC_Info/1
  [DTC_clear_request] -> DTC_Info/4
  VPMM_PowerUpState_enum/1 -> [VPMM_PowerUpState_enum]

== system ddm/DDM/DDM/PMM/power up and power down/DCDC ready for precharge fail ==
  note: Diagnostics and Fault Handling
  note: Test Detection Criteria
  note: Release Condition After Decision
  note: Test Pass Criteria
  task_time_s : Inport
  VPMM_PowerSta_enum : Inport  Port=2
  VPMM_PwrStaSW_enum : Inport  Port=3
  VINP_DCDCReady4Pre_flg : Inport  Port=4
  VPMM_PowerUpFault_enum : Inport  Port=5
  VINP_ReqClrDTC_flg : Inport  Port=6
  VPMM_PowerUpState_enum : Inport  Port=7
  Constant : Constant  Value=ENUM_PUFAULT_PRECHRGCHKFAIL
  Constant12 : Constant  Value=ENUM_PWRSTASW_OFF
  Constant13 : Constant  Value=FALSE
  Constant14 : Constant  Value=ZERO_INT
  Constant17 : Constant  Value=KDDM_PwrUpDnDiagnosisOffSW_flg
  Constant18 : Constant  Value=KDDM_DCDC4PrePassTO_s
  Constant22 : Constant  Value=ENUM_POWERSTA_OFF
  Constant28 : Constant  Value=KDDM_DCDC4PrePassTO_s
  Constant29 : Constant  Value=FALSE
  Constant3 : Constant  Value=KDDM_DCDC4PreDTC_cnt
  Constant4 : Constant  Value=FALSE
  Constant41 : Constant  Value=KDDM_DCDC4PreDetTO_s
  Constant5 : Constant  Value=ENUM_PUSTATE_COMPLETED
  Constant6 : Constant  Value=TRUE
  Constant7 : Constant  Value=ENUM_POWERSTA_STANDBY
  Constant9 : Constant  Value=KDDM_DCDC4PreDTC_cnt
  DTC_Couter1 : hcu_lib/Basic_Blocks/DTC_Couter
  DTC_Info : hcu_lib/Basic_Blocks/DTC_Info
  Equal{1,3,8..9} (4 alike) : RelationalOperator  Operator===  OutDataTypeStr=boolean  RndMeth=Simplest
  Equal4 : RelationalOperator  Operator=~=  OutDataTypeStr=boolean  RndMeth=Simplest
  Equal7 : RelationalOperator  OutDataTypeStr=boolean  RndMeth=Simplest
  Logical Operator13 : Logic  Operator=NOT  AllPortsSameDT=off  OutDataTypeStr=boolean
  Logical Operator14 : Logic  Operator=OR  Inputs=4  AllPortsSameDT=off  OutDataTypeStr=boolean
  Logical Operator16 : Logic  AllPortsSameDT=off  OutDataTypeStr=boolean
  Logical Operator4 : Logic  Operator=NOT  AllPortsSameDT=off  OutDataTypeStr=boolean
  Logical Operator5 : Logic  AllPortsSameDT=off  OutDataTypeStr=boolean
  Relational Operator1 : RelationalOperator  Operator=>  OutDataTypeStr=boolean  RndMeth=Simplest
  Switch1 : Switch  Criteria=u2 ~= 0
  Switch3 : Switch  Criteria=u2 ~= 0
  Switch6 : Switch  Criteria=u2 ~= 0
  Terminator : Terminator
  Test Detection Criteria1 : hcu_lib/Basic_Blocks/Test Detection Criteria
  Timer2 : hcu_lib/Basic_Blocks/Timer
  Unit Delay1 : UnitDelay  SampleTime=-1  HasFrameUpgradeWarning=on
  VDDM_DCDC4PreDTC_raw32 : Outport
  VDDM_DCDC4PreCFS_flg : Outport  Port=2
  wires:
  [VDDM_DCDC4PreCFS_flg] -> VDDM_DCDC4PreCFS_flg/1
  Logical Operator13/1 -> Timer2/1
  [VDDM_DCDC4PreChk_flg] -> Switch3/1
  Constant17/1 -> Logical Operator14/4
  Constant28/1 -> Equal7/2
  [VDDM_DCDC4PreCFSRls_flg] -> Switch6/2
  Constant3/1 -> DTC_Couter1/3
  Equal7/1 -> [VDDM_DCDC4PrePass_flg]  "VDDM_DCDC4PrePass_flg"
  Relational Operator1/1 -> Terminator/1  "VDDM_DCDC4PreDFS_flg"
  Logical Operator14/1 -> [VDDM_DCDC4PreCFSRls_flg]  "VDDM_DCDC4PreCFSRls_flg"
  Equal8/1 -> Logical Operator16/1
  DTC_Couter1/1 -> [VDDM_DCDC4PreCFS_flg]  "VDDM_DCDC4PreCFS_flg"
  [VDDM_DCDC4PreDet_flg] -> DTC_Couter1/1
  Constant41/1 -> Test Detection Criteria1/4
  Constant4/1 -> Switch1/1
  [VPMM_PowerUpState_enum] -> Equal3/1
  [VPMM_PwrStaSW_enum] -> Equal4/1
  Constant13/1 -> Switch3/3
  Timer2/1 -> Equal7/1
  Logical Operator16/1 -> Logical Operator14/1
  Constant6/1 -> Switch1/3
  [VDDM_DCDC4PrePass_flg] -> Logical Operator14/3
  Constant12/1 -> Equal4/2
  Equal3/1 -> Switch1/2
  Switch1/1 -> Logical Operator13/1, Timer2/2
  Constant14/1 -> Relational Operator1/2
  Switch3/1 -> Switch6/3
  [DTC_clear_request] -> Logical Operator14/2
  Constant29/1 -> Switch6/1
  Constant5/1 -> Equal3/2
  Equal4/1 -> Switch3/2
  [VPMM_PowerSta_enum] -> Equal9/1
  Constant7/1 -> Equal9/2
  [VDDM_DCDC4PreCFSRls_flg] -> DTC_Couter1/2
  Unit Delay1/1 -> Equal8/1
  [task_time_s] -> Test Detection Criteria1/2
  Equal9/1 -> Logical Operator16/2
  Switch6/1 -> Test Detection Criteria1/1
  Constant9/1 -> Test Detection Criteria1/3
  [task_time_s] -> Timer2/3
  [VPMM_PowerSta_enum] -> Unit Delay1/1
  Constant22/1 -> Equal8/2
  DTC_Couter1/2 -> Relational Operator1/1  "VDDM_DCDC4PreDTC_cnt"
  Test Detection Criteria1/1 -> [VDDM_DCDC4PreDet_flg]  "VDDM_DCDC4PreDet_flg"
  Constant18/1 -> Timer2/4
  VPMM_PowerSta_enum/1 -> [VPMM_PowerSta_enum]
  VPMM_PwrStaSW_enum/1 -> [VPMM_PwrStaSW_enum]
  task_time_s/1 -> [task_time_s]
  VINP_ReqClrDTC_flg/1 -> [DTC_clear_request]
  Equal1/1 -> Logical Operator5/2
  Constant/1 -> Equal1/2
  VPMM_PowerUpFault_enum/1 -> Equal1/1
  Logical Operator5/1 -> [VDDM_DCDC4PreChk_flg]
  VINP_DCDCReady4Pre_flg/1 -> Logical Operator4/1
  Logical Operator4/1 -> Logical Operator5/1
  DTC_Info/1 -> VDDM_DCDC4PreDTC_raw32/1  "VDDM_DCDC4PreDTC_raw32"
  [VDDM_DCDC4PrePass_flg] -> DTC_Info/2
  [VDDM_DCDC4PreCFS_flg] -> DTC_Info/3
  [VDDM_DCDC4PreDet_flg] -> DTC_Info/1
  [DTC_clear_request] -> DTC_Info/4
  VPMM_PowerUpState_enum/1 -> [VPMM_PowerUpState_enum]

== system ddm/DDM/DDM/PMM/power up and power down/HVB ready for precharge fail ==
  note: Diagnostics and Fault Handling
  note: Release Condition After Decision
  note: Test Detection Criteria
  note: Test Pass Criteria
  task_time_s : Inport
  VPMM_PowerSta_enum : Inport  Port=2
  VPMM_PwrStaSW_enum : Inport  Port=3
  VINP_HVBattReady4Pre_enum : Inport  Port=4
  VPMM_PowerUpFault_enum : Inport  Port=5
  DTC_clear_request : Inport  Port=6
  VPMM_PowerUpState_enum : Inport  Port=7
  Constant : Constant  Value=ENUM_PUFAULT_PRECHRGCHKFAIL
  Constant1 : Constant  Value=FALSE
  Constant12 : Constant  Value=ENUM_PWRSTASW_OFF
  Constant13 : Constant  Value=FALSE
  Constant17 : Constant  Value=KDDM_PwrUpDnDiagnosisOffSW_flg
  Constant18 : Constant  Value=KDDM_HVB4PreDTC_cnt
  Constant2 : Constant  Value=ENUM_PUSTATE_COMPLETED
  Constant22 : Constant  Value=ENUM_POWERSTA_OFF
  Constant23 : Constant  Value=TRUE
  Constant28 : Constant  Value=KDDM_HVB4PrePassTO_s
  Constant3 : Constant  Value=ENUM_HVBATTREADYPRE_READY
  Constant4 : Constant  Value=ENUM_POWERSTA_STANDBY
  Constant40 : Constant  Value=KDDM_HVB4PreDTC_cnt
  Constant41 : Constant  Value=KDDM_HVB4PreDetTO_s
  Constant5 : Constant  Value=ZERO_INT
  Constant7 : Constant  Value=KDDM_HVB4PrePassTO_s
  Constant9 : Constant  Value=FALSE
  DTC_Couter1 : hcu_lib/Basic_Blocks/DTC_Couter
  DTC_Info : hcu_lib/Basic_Blocks/DTC_Info
  Equal{1,7..9} (4 alike) : RelationalOperator  Operator===  OutDataTypeStr=boolean  RndMeth=Simplest
  Equal2 : RelationalOperator  Operator=~=  OutDataTypeStr=boolean  RndMeth=Simplest
  Equal24 : RelationalOperator  Operator=~=  OutDataTypeStr=boolean  RndMeth=Simplest
  Equal6 : RelationalOperator  OutDataTypeStr=boolean  RndMeth=Simplest
  Logical Operator13 : Logic  Operator=NOT  AllPortsSameDT=off  OutDataTypeStr=boolean
  Logical Operator14 : Logic  Operator=OR  Inputs=4  AllPortsSameDT=off  OutDataTypeStr=boolean
  Logical Operator16 : Logic  AllPortsSameDT=off  OutDataTypeStr=boolean
  Logical Operator4 : Logic  AllPortsSameDT=off  OutDataTypeStr=boolean
  Relational Operator1 : RelationalOperator  Operator=>  OutDataTypeStr=boolean  RndMeth=Simplest
  Switch2 : Switch  Criteria=u2 ~= 0
  Switch3 : Switch  Criteria=u2 ~= 0
  Switch6 : Switch  Criteria=u2 ~= 0
  Terminator : Terminator
  Test Detection Criteria : hcu_lib/Basic_Blocks/Test Detection Criteria
  Timer2 : hcu_lib/Basic_Blocks/Timer
  Unit Delay1 : UnitDelay  SampleTime=-1  HasFrameUpgradeWarning=on
  VDDM_HVB4PreDTC_raw32 : Outport
  VDDM_HVB4PreCFS_flg : Outport  Port=2
  wires:
  [VDDM_HVB4PreCFS_flg] -> VDDM_HVB4PreCFS_flg/1
  Constant1/1 -> Switch2/1
  [VPMM_PowerUpState_enum] -> Equal1/1
  Equal1/1 -> Switch2/2
  Constant2/1 -> Equal1/2
  Constant23/1 -> Switch2/3
  [VPMM_PwrStaSW_enum] -> Equal2/1
  Constant12/1 -> Equal2/2
  [task_time_s] -> Test Detection Criteria/2
  Switch3/1 -> Switch6/3
  Logical Operator13/1 -> Timer2/1
  Constant28/1 -> Timer2/4
  DTC_Couter1/1 -> [VDDM_HVB4PreCFS_flg]  "VDDM_HVB4PreCFS_flg"
  Equal6/1 -> [VDDM_HVB4PrePass_flg]  "VDDM_HVB4PrePass_flg"
  [DTC_clear_request] -> Logical Operator14/2
  [VPMM_PowerSta_enum] -> Unit Delay1/1
  Constant40/1 -> Test Detection Criteria/3
  [VDDM_HVB4PreChk_flg] -> Switch3/1
  Equal2/1 -> Switch3/2
  Switch2/1 -> Logical Operator13/1, Timer2/2
  [VPMM_PowerSta_enum] -> Equal9/1
  Test Detection Criteria/1 -> [VDDM_HVB4PreDet_flg]  "VDDM_HVB4PreDet_flg"
  Unit Delay1/1 -> Equal7/1
  Logical Operator16/1 -> Logical Operator14/1
  Equal7/1 -> Logical Operator16/1
  Switch6/1 -> Test Detection Criteria/1
  Constant17/1 -> Logical Operator14/4
  [task_time_s] -> Timer2/3
  Logical Operator14/1 -> [VDDM_HVB4PreCFSRls_flg]  "VDDM_HVB4PreCFSRls_flg"
  Constant13/1 -> Switch3/3
  [VDDM_HVB4PrePass_flg] -> Logical Operator14/3
  Constant4/1 -> Equal9/2
  Constant5/1 -> Relational Operator1/2
  Equal9/1 -> Logical Operator16/2
  Constant18/1 -> DTC_Couter1/3
  Constant22/1 -> Equal7/2
  [VDDM_HVB4PreCFSRls_flg] -> DTC_Couter1/2
  Relational Operator1/1 -> Terminator/1  "VDDM_HVB4PreDFS_flg"
  DTC_Couter1/2 -> Relational Operator1/1  "VDDM_HVB4PreDTC_cnt"
  Constant9/1 -> Switch6/1
  [VDDM_HVB4PreCFSRls_flg] -> Switch6/2
  Constant41/1 -> Test Detection Criteria/4
  [VDDM_HVB4PreDet_flg] -> DTC_Couter1/1
  Timer2/1 -> Equal6/1
  Constant7/1 -> Equal6/2
  VPMM_PowerSta_enum/1 -> [VPMM_PowerSta_enum]
  VPMM_PwrStaSW_enum/1 -> [VPMM_PwrStaSW_enum]
  task_time_s/1 -> [task_time_s]
  Constant3/1 -> Equal24/2
  VINP_HVBattReady4Pre_enum/1 -> Equal24/1
  DTC_clear_request/1 -> [DTC_clear_request]
  Constant/1 -> Equal8/2
  VPMM_PowerUpFault_enum/1 -> Equal8/1
  Equal24/1 -> Logical Operator4/1
  Equal8/1 -> Logical Operator4/2
  Logical Operator4/1 -> [VDDM_HVB4PreChk_flg]
  DTC_Info/1 -> VDDM_HVB4PreDTC_raw32/1  "VDDM_HVB4PreDTC_raw32"
  [VDDM_HVB4PreCFS_flg] -> DTC_Info/3
  [VDDM_HVB4PrePass_flg] -> DTC_Info/2
  [VDDM_HVB4PreDet_flg] -> DTC_Info/1
  [DTC_clear_request] -> DTC_Info/4
  VPMM_PowerUpState_enum/1 -> [VPMM_PowerUpState_enum]

== system ddm/DDM/DDM/PMM/power up and power down/High level system safety check fail ==
  note: Diagnostics and Fault Handling
  note: Test Detection Criteria
  note: Release Condition After Decision
  note: Test Pass Criteria
  task_time_s : Inport
  VPMM_PowerSta_enum : Inport  Port=2
  VPMM_PwrStaSW_enum : Inport  Port=3
  VPMM_SafetyChkHLv_flg : Inport  Port=4
  VPMM_PowerUpFault_enum : Inport  Port=5
  DTC_clear_request : Inport  Port=6
  VPMM_PowerUpState_enum : Inport  Port=7
  Constant : Constant  Value=ENUM_PUFAULT_SAFETYCHKFAIL
  Constant12 : Constant  Value=ENUM_PWRSTASW_OFF
  Constant13 : Constant  Value=FALSE
  Constant14 : Constant  Value=ZERO_INT
  Constant17 : Constant  Value=KDDM_PwrUpDnDiagnosisOffSW_flg
  Constant18 : Constant  Value=KDDM_HiLvSaChkPassTO_s
  Constant22 : Constant  Value=ENUM_POWERSTA_OFF
  Constant28 : Constant  Value=KDDM_HiLvSaChkPassTO_s
  Constant29 : Constant  Value=FALSE
  Constant3 : Constant  Value=KDDM_HiLvSaChkDTC_cnt
  Constant4 : Constant  Value=FALSE
  Constant41 : Constant  Value=KDDM_HiLvSaChkDetTO_s
  Constant5 : Constant  Value=ENUM_PUSTATE_COMPLETED
  Constant6 : Constant  Value=TRUE
  Constant7 : Constant  Value=ENUM_POWERSTA_STANDBY
  Constant9 : Constant  Value=KDDM_HiLvSaChkDTC_cnt
  DTC_Couter1 : hcu_lib/Basic_Blocks/DTC_Couter
  DTC_Info : hcu_lib/Basic_Blocks/DTC_Info
  Equal{1,3,8..9} (4 alike) : RelationalOperator  Operator===  OutDataTypeStr=boolean  RndMeth=Simplest
  Equal4 : RelationalOperator  Operator=~=  OutDataTypeStr=boolean  RndMeth=Simplest
  Equal7 : RelationalOperator  OutDataTypeStr=boolean  RndMeth=Simplest
  Logical Operator13 : Logic  Operator=NOT  AllPortsSameDT=off  OutDataTypeStr=boolean
  Logical Operator14 : Logic  Operator=OR  Inputs=4  AllPortsSameDT=off  OutDataTypeStr=boolean
  Logical Operator16 : Logic  AllPortsSameDT=off  OutDataTypeStr=boolean
  Logical Operator4 : Logic  Operator=NOT  AllPortsSameDT=off  OutDataTypeStr=boolean
  Logical Operator5 : Logic  AllPortsSameDT=off  OutDataTypeStr=boolean
  Relational Operator1 : RelationalOperator  Operator=>  OutDataTypeStr=boolean  RndMeth=Simplest
  Switch1 : Switch  Criteria=u2 ~= 0
  Switch3 : Switch  Criteria=u2 ~= 0
  Switch6 : Switch  Criteria=u2 ~= 0
  Terminator : Terminator
  Test Detection Criteria1 : hcu_lib/Basic_Blocks/Test Detection Criteria
  Timer2 : hcu_lib/Basic_Blocks/Timer
  Unit Delay1 : UnitDelay  SampleTime=-1  HasFrameUpgradeWarning=on
  VDDM_HiLvSaChkDTC_raw32 : Outport
  VDDM_HiLvSaChkCFS_flg : Outport  Port=2
  wires:
  [VDDM_HiLvSaChkCFS_flg] -> VDDM_HiLvSaChkCFS_flg/1
  Equal4/1 -> Switch3/2
  Constant9/1 -> Test Detection Criteria1/3
  Logical Operator14/1 -> [VDDM_HiLvSaChkCFSRls_flg]  "VDDM_HiLvSaChkCFSRls_flg"
  Logical Operator16/1 -> Logical Operator14/1
  Constant28/1 -> Equal7/2
  Constant3/1 -> DTC_Couter1/3
  Constant18/1 -> Timer2/4
  [VDDM_HiLvSaChkChk_flg] -> Switch3/1
  DTC_Couter1/1 -> [VDDM_HiLvSaChkCFS_flg]  "VDDM_HiLvSaChkCFS_flg"
  Test Detection Criteria1/1 -> [VDDM_HiLvSaChkDet_flg]  "VDDM_HiLvSaChkDet_flg"
  Constant41/1 -> Test Detection Criteria1/4
  [VDDM_HiLvSaChkCFSRls_flg] -> DTC_Couter1/2
  [VDDM_HiLvSaChkCFSRls_flg] -> Switch6/2
  [VDDM_HiLvSaChkDet_flg] -> DTC_Couter1/1
  Equal3/1 -> Switch1/2
  Constant12/1 -> Equal4/2
  Equal8/1 -> Logical Operator16/1
  Logical Operator13/1 -> Timer2/1
  Constant17/1 -> Logical Operator14/4
  [task_time_s] -> Timer2/3
  DTC_Couter1/2 -> Relational Operator1/1  "VDDM_HiLvSaChkDTC_cnt"
  Switch6/1 -> Test Detection Criteria1/1
  [VPMM_PowerSta_enum] -> Unit Delay1/1
  Timer2/1 -> Equal7/1
  [VPMM_PowerSta_enum] -> Equal9/1
  Constant22/1 -> Equal8/2
  Unit Delay1/1 -> Equal8/1
  Equal9/1 -> Logical Operator16/2
  Constant5/1 -> Equal3/2
  Constant7/1 -> Equal9/2
  Equal7/1 -> [VDDM_HiLvSaChkPass_flg]  "VDDM_HiLvSaChkPass_flg"
  Constant14/1 -> Relational Operator1/2
  [task_time_s] -> Test Detection Criteria1/2
  Constant29/1 -> Switch6/1
  Switch3/1 -> Switch6/3
  Switch1/1 -> Logical Operator13/1, Timer2/2
  [DTC_clear_request] -> Logical Operator14/2
  Constant13/1 -> Switch3/3
  [VDDM_HiLvSaChkPass_flg] -> Logical Operator14/3
  Constant6/1 -> Switch1/3
  [VPMM_PwrStaSW_enum] -> Equal4/1
  [VPMM_PowerUpState_enum] -> Equal3/1
  Constant4/1 -> Switch1/1
  Relational Operator1/1 -> Terminator/1  "VDDM_HiLvSaChkDFS_flg"
  Logical Operator5/1 -> [VDDM_HiLvSaChkChk_flg]
  VPMM_PowerUpFault_enum/1 -> Equal1/1
  VPMM_SafetyChkHLv_flg/1 -> Logical Operator4/1
  Logical Operator4/1 -> Logical Operator5/1
  Equal1/1 -> Logical Operator5/2
  Constant/1 -> Equal1/2
  DTC_clear_request/1 -> [DTC_clear_request]
  VPMM_PowerSta_enum/1 -> [VPMM_PowerSta_enum]
  VPMM_PwrStaSW_enum/1 -> [VPMM_PwrStaSW_enum]
  task_time_s/1 -> [task_time_s]
  DTC_Info/1 -> VDDM_HiLvSaChkDTC_raw32/1  "VDDM_HiLvSaChkDTC_raw32"
  [VDDM_HiLvSaChkPass_flg] -> DTC_Info/2
  [VDDM_HiLvSaChkCFS_flg] -> DTC_Info/3
  [VDDM_HiLvSaChkDet_flg] -> DTC_Info/1
  [DTC_clear_request] -> DTC_Info/4
  VPMM_PowerUpState_enum/1 -> [VPMM_PowerUpState_enum]
